simulink model "mainModels"  (R2017b)
settings: Solver=FixedStepAuto  StartTime=0.0  StopTime=3  FixedStep=1e-2  RelTol=1e-3
values from neighbouring files (symbols this model uses):
  A1 = [0 1 0 0 ... (first row only)    [calcSystem.m]
  B1 = [0 ... (first row only)    [calcSystem.m]
  C1 = [1 0 0 0 ... (first row only)    [calcSystem.m]
  D1 = [0 ... (first row only)    [calcSystem.m]
settings Model: Creator=Haotian  LastModifiedBy=Haotian

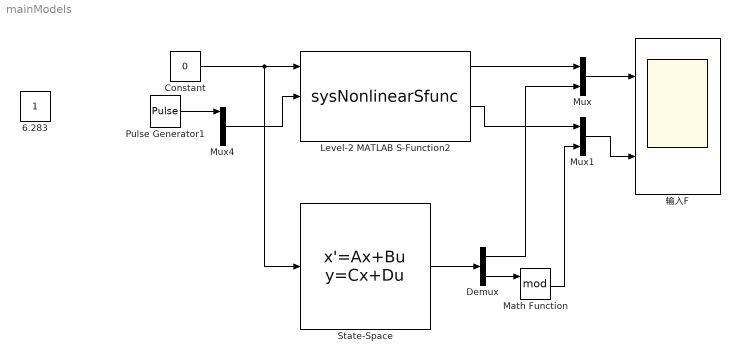
== system mainModels ==
  Constant : Constant  Value=0
  Demux : Demux  Outputs=2
  Level-2 MATLAB S-Function2 : M-S-Function  FunctionName=sysNonlinearSfunc  Parameters=Mc, Mg, b, l, I, init_phi, useAcc  mask(S-function: sysNonlinearSfunc){Mc=1.096, Mg=0.109, b=0.1, l=0.25, I=0.0034, init_phi=0.01, useAcc=on}
      mask prompts: Mc "小车质量"; Mg "摆杆质量"; b "小车摩擦系数"; l "摆杆转动轴心到杆质心的长度"; I "摆杆惯量"; init_phi "初始垂直夹角"; useAcc "使用加速度作为输入"
      mask help: 一阶倒立摆非线性模型。
      mask Display:
      | fprintf('一阶倒立摆\n\nM=%.3f m=%.3f\nb=%.3f l=%.3f\nI=%.3f phi0=%.2f\n\nX=[x dx phi dphi]', Mc, Mg, b, l, I, init_phi);
      | if(useAcc)
      |     port_label('input', 1, 'a');
      | else
      |     port_label('input', 1, 'F');
      | end
      | port_label('input', 2, 'setX');
      | port_label('input', 3, 'devX');
      | 
      | port_label('output', 1, 'x');
      | port_label('output', 2, 'v');
      | port_label('output', 3, '\phi','texmode','on');
      | port_label('output', 4, 'd\phi','texmode','on');
  Math Function : Math  Operator=mod  SaturateOnIntegerOverflow=on
  Mux : Mux  Inputs=2
  Mux1 : Mux  Inputs=2
  Mux4 : Mux
  Pulse Generator1 : DiscretePulseGenerator  PulseType=Time based  Period=10  PhaseDelay=1
  State-Space : StateSpace  A=A1  B=B1  C=C1  D=D1  InitialCondition=[0 0 0.01 0]
  输入F : Scope  NumInputPorts=2
  6.283 : Constant  IOType=siggen
  wires:
  Constant/1 -> Level-2 MATLAB S-Function2/1, State-Space/1
  State-Space/1 -> Demux/1
  Level-2 MATLAB S-Function2/3 -> Mux1/1
  Demux/2 -> Math Function/1
  Mux1/1 -> 输入F/2
  Mux/1 -> 输入F/1
  Level-2 MATLAB S-Function2/1 -> Mux/1
  Math Function/1 -> Mux1/2
  Demux/1 -> Mux/2
  Pulse Generator1/1 -> Mux4/1
  Mux4/1 -> Level-2 MATLAB S-Function2/2
